simulink model "PIDFrac"  (R2022b)
settings: Solver=FixedStepAuto  StartTime=0.0  StopTime=60  FixedStep=Ts  RelTol=1e-3
values from neighbouring files (symbols this model uses):
  g = 9.81    [PIDarbitrario.m]
  kdc = 0.334436620011803    (= 0.334436620012)    [PIDarbitrario.m]
  kdp = -15.864761054699    (= -15.8647610547)    [PIDarbitrario.m]
  kic = 0.00199754552839596    (= 0.0019975455284)    [PIDarbitrario.m]
  kip = -3726.07419650531    (= -3726.07419651)    [PIDarbitrario.m]
  kpc = 0.0704426191079745    (= 0.070442619108)    [PIDarbitrario.m]
  kpp = -556.27969825542    (= -556.279698255)    [PIDarbitrario.m]
  L = 0.25    [PIDarbitrario.m]
  m = 0.03    [PIDarbitrario.m]
  M = 0.510    (= 0.51)    [PIDarbitrario.m]
  Ts = 0.010    (= 0.01)    [PIDarbitrario.m]
  ts = 5    [PIDarbitrario.m]
undefined symbols (not defined in the file or in its folder): Ddc, Ddp, Dic, Dip, Ndc, Ndp, Nic, Nip
libraries: spsStairGeneratorLib x1
settings Model: Creator=manue  LastModifiedBy=manue

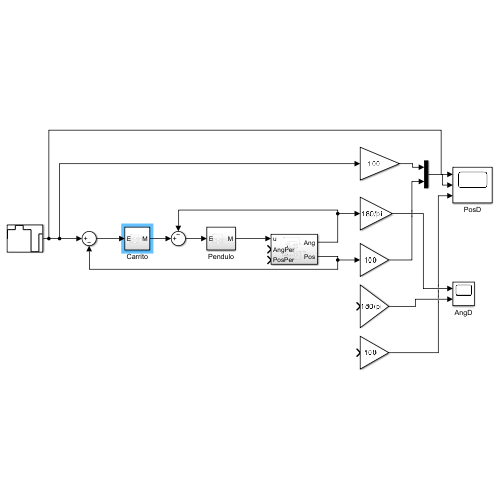
[thumbnail: Simulink's stored preview of the top-level diagram]
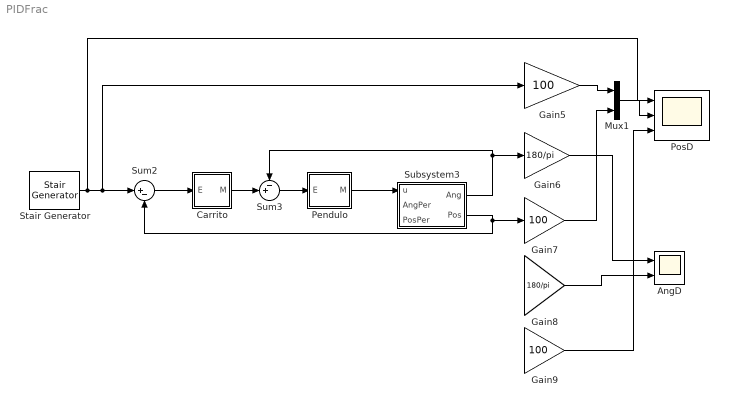
== system PIDFrac ==
  AngD : Scope  NumInputPorts=2
  Carrito : Subsystem
  Gain5 : Gain  Gain=100
  Gain6 : Gain  Gain=180/pi
  Gain7 : Gain  Gain=100
  Gain8 : Gain  Gain=180/pi
  Gain9 : Gain  Gain=100
  Mux1 : Mux  Inputs=2
  Pendulo : Subsystem
  PosD : Scope  NumInputPorts=3
  Stair Generator : spsStairGeneratorLib/Stair Generator  t=[0, ts,2*ts,3*ts,4*ts,5*ts,6*ts,7*ts,8*ts,9*ts,10*ts]  e=[25,35,35,40,40,35,35,10,10,30,30]/100  Ts=Ts
  Subsystem3 : Subsystem
  Sum2 : Sum  Inputs=|+-
  Sum3 : Sum  Inputs=-+|
  wires:
  Subsystem3/2(Pos) -> Gain7/1, Sum2/2
  Stair Generator/1 -> PosD/1, Gain5/1, Sum2/1
  Gain6/1 -> AngD/1
  Gain5/1 -> Mux1/1
  Mux1/1 -> PosD/2
  Gain8/1 -> AngD/2
  Gain9/1 -> PosD/3
  Sum2/1 -> Carrito/1(E)
  Gain7/1 -> Mux1/2
  Carrito/1(M) -> Sum3/2
  Subsystem3/1(Ang) -> Sum3/1, Gain6/1
  Pendulo/1(M) -> Subsystem3/1(u)
  Sum3/1 -> Pendulo/1(E)

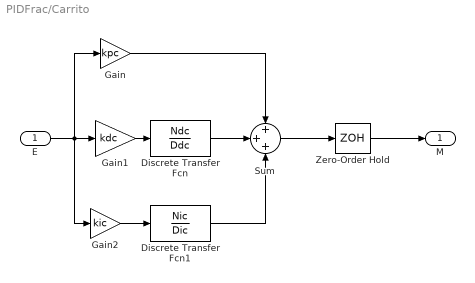
== system PIDFrac/Carrito ==
  E : Inport
  Discrete Transfer Fcn : DiscreteTransferFcn  Numerator=Ndc  Denominator=Ddc  SampleTime=Ts
  Discrete Transfer Fcn1 : DiscreteTransferFcn  Numerator=Nic  Denominator=Dic  SampleTime=Ts
  Gain : Gain  Gain=kpc
  Gain1 : Gain  Gain=kdc
  Gain2 : Gain  Gain=kic
  Sum : Sum  Inputs=+++
  Zero-Order Hold : ZeroOrderHold  SampleTime=Ts
  M : Outport
  wires:
  Discrete Transfer Fcn/1 -> Sum/2
  Discrete Transfer Fcn1/1 -> Sum/3
  Gain/1 -> Sum/1
  Sum/1 -> Zero-Order Hold/1
  Zero-Order Hold/1 -> M/1
  E/1 -> Gain2/1, Gain1/1, Gain/1
  Gain1/1 -> Discrete Transfer Fcn/1
  Gain2/1 -> Discrete Transfer Fcn1/1

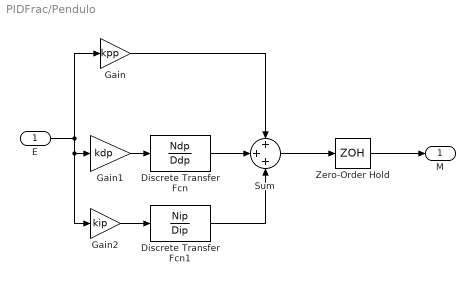
== system PIDFrac/Pendulo ==
  E : Inport
  Discrete Transfer Fcn : DiscreteTransferFcn  Numerator=Ndp  Denominator=Ddp  SampleTime=Ts
  Discrete Transfer Fcn1 : DiscreteTransferFcn  Numerator=Nip  Denominator=Dip  SampleTime=Ts
  Gain : Gain  Gain=kpp
  Gain1 : Gain  Gain=kdp
  Gain2 : Gain  Gain=kip
  Sum : Sum  Inputs=+++
  Zero-Order Hold : ZeroOrderHold  SampleTime=Ts
  M : Outport
  wires:
  Discrete Transfer Fcn/1 -> Sum/2
  Zero-Order Hold/1 -> M/1
  E/1 -> Gain2/1, Gain1/1, Gain/1
  Sum/1 -> Zero-Order Hold/1
  Gain/1 -> Sum/1
  Discrete Transfer Fcn1/1 -> Sum/3
  Gain1/1 -> Discrete Transfer Fcn/1
  Gain2/1 -> Discrete Transfer Fcn1/1

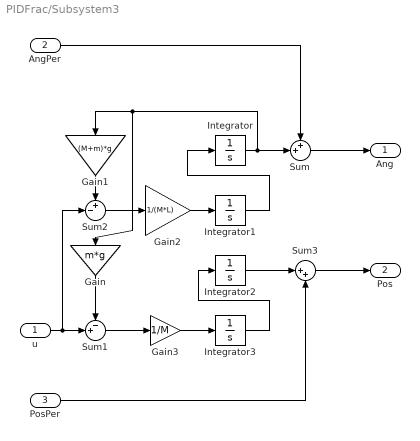
== system PIDFrac/Subsystem3 ==
  u : Inport
  AngPer : Inport  Port=2
  PosPer : Inport  Port=3
  Gain : Gain  Gain=m*g
  Gain1 : Gain  Gain=(M+m)*g
  Gain2 : Gain  Gain=1/(M*L)
  Gain3 : Gain  Gain=1/M
  Integrator : Integrator  InitialCondition=10*pi/180
  Integrator1 : Integrator
  Integrator2 : Integrator
  Integrator3 : Integrator
  Sum : Sum  Inputs=++|
  Sum1 : Sum  Inputs=-+|
  Sum2 : Sum  Inputs=+-|
  Sum3 : Sum  Inputs=|++
  Ang : Outport
  Pos : Outport  Port=2
  wires:
  AngPer/1 -> Sum/1
  Integrator/1 -> Gain1/1, Gain/1, Sum/2
  Gain/1 -> Sum1/1
  Gain1/1 -> Sum2/1
  u/1 -> Sum2/2, Sum1/2
  Sum2/1 -> Gain2/1
  Gain2/1 -> Integrator1/1
  Integrator1/1 -> Integrator/1
  Sum1/1 -> Gain3/1
  Gain3/1 -> Integrator3/1
  Integrator3/1 -> Integrator2/1
  Integrator2/1 -> Sum3/1
  PosPer/1 -> Sum3/2
  Sum3/1 -> Pos/1
  Sum/1 -> Ang/1
